simulink subsystem "Axial_Drag"  (R2024b)
settings: Solver=VariableStepAuto  StartTime=0.0  StopTime=10.0  RelTol=1e-3
values from neighbouring files (symbols this model uses):
  Ar = 0.0181458391671    [barrowaman.mat]
  CD_data = [0.45 0.45 0.45 0.45 0.45 0.45 0.45 0.45 0.45 0.45 0.45 0.45 ... (664 elements, 664x1)]    [barrowaman.mat]
  CD_input = [0.0002927 0.0003023 0.0003533 0.0009319 0.003 0.007 0.01 0.014 0.018 0.022 0.025 0.029 ... (664 elements, 664x1)]    [barrowaman.mat]
settings Model: Creator=joedo  LastModifiedBy=joedo

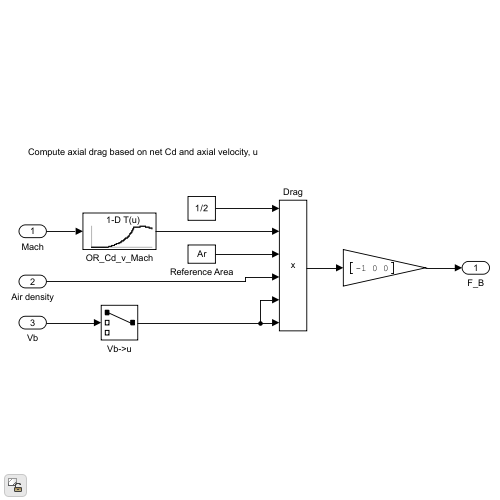
[thumbnail: Simulink's stored preview of the top-level diagram]
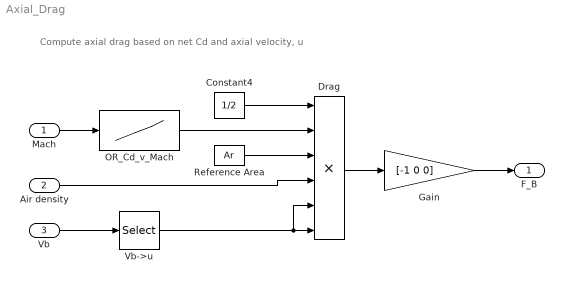
== system Axial_Drag ==
  note: Compute axial drag based on net Cd and axial velocity, u
  Mach : Inport
  Air density : Inport  Port=2
  Vb : Inport  Port=3
  Constant4 : Constant  Value=1/2
  Drag : Product  Inputs=6
  Gain : Gain  Gain=[-1 0 0]
  OR_Cd_v_Mach : Lookup_n-D  NumberOfTableDimensions=1  BreakpointsForDimension1=CD_input  Table=CD_data  InternalRulePriority=Speed  RndMeth=Simplest
  Reference Area : Constant  Value=Ar
  Vb->u : Selector  InputPortWidth=3  IndexOptions=Index vector (dialog)  Indices=[1]  OutputSizes=1
  F_B : Outport  VectorParamsAs1DForOutWhenUnconnected=off
  wires:
  Mach/1 -> OR_Cd_v_Mach/1
  Gain/1 -> F_B/1
  Drag/1 -> Gain/1
  Constant4/1 -> Drag/1
  OR_Cd_v_Mach/1 -> Drag/2
  Vb/1 -> Vb->u/1
  Vb->u/1 -> Drag/5, Drag/6
  Air density/1 -> Drag/4
  Reference Area/1 -> Drag/3
